simulink model "day03"  (R2026a)
settings: Solver=VariableStepAuto  StopTime=inf
libraries: simulink x1
settings Model: Creator=pete  LastModifiedBy=pete

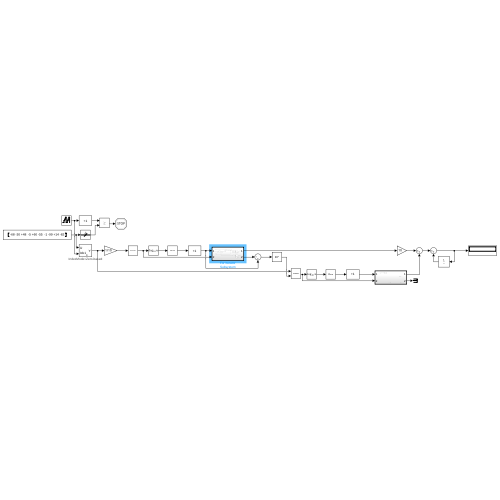
[thumbnail: Simulink's stored preview of the top-level diagram]
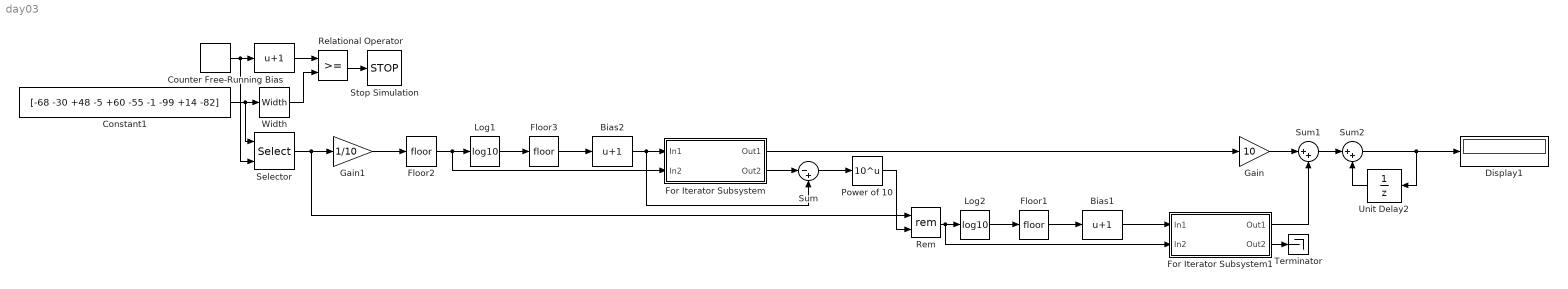
== system day03 ==
  Bias : Bias  Bias=1  SaturateOnIntegerOverflow=off
  Bias1 : Bias  Bias=1  SaturateOnIntegerOverflow=off
  Bias2 : Bias  Bias=1  SaturateOnIntegerOverflow=off
  Constant1 : Constant  Value=[-68 -30 +48 -5 +60 -55 -1 -99 +14 -82]
  Counter Free-Running : simulink/Sources/Counter Free-Running  NumBits=16  tsamp=-1
  Display1 : Display
  Floor1 : Rounding
  Floor2 : Rounding
  Floor3 : Rounding
  For Iterator Subsystem : Subsystem  TreatAsAtomicUnit=on
  For Iterator Subsystem1 : Subsystem  TreatAsAtomicUnit=on
  Gain : Gain  Gain=10
  Gain1 : Gain  Gain=1/10
  Log1 : Math  Operator=log10
  Log2 : Math  Operator=log10
  Power of 10 : Math  Operator=10^u
  Relational Operator : RelationalOperator  OutDataTypeStr=boolean  RndMeth=Simplest  InputSameDT=off
  Rem : Math  Operator=rem
  Selector : Selector  IndexMode=Zero-based  InputPortWidth=10  IndexOptions=Index vector (port)  Indices=[1 3]  OutputSizes=1
      settings: AttributesFormatString=IndexMode=%<IndexMode>
  Stop Simulation : Stop
  Sum : Sum  Inputs=|-+
  Sum1 : Sum  Inputs=|++
  Sum2 : Sum  Inputs=|++
  Terminator : Terminator
  Unit Delay2 : UnitDelay  SampleTime=-1
  Width : Width
  wires:
  Counter Free-Running/1 -> Selector/2, Bias/1
  Bias/1 -> Relational Operator/1
  Relational Operator/1 -> Stop Simulation/1
  Width/1 -> Relational Operator/2
  Constant1/1 -> Selector/1, Width/1
  Unit Delay2/1 -> Sum2/2
  Sum2/1 -> Display1/1, Unit Delay2/1
  Gain1/1 -> Floor2/1
  Log1/1 -> Floor3/1
  Floor3/1 -> Bias2/1
  Floor2/1 -> For Iterator Subsystem/2(In2), Log1/1
  Selector/1 -> Rem/1, Gain1/1
  Bias2/1 -> Sum/2, For Iterator Subsystem/1(In1)
  For Iterator Subsystem/2(Out2) -> Sum/1
  Sum/1 -> Power of 10/1
  Power of 10/1 -> Rem/2
  Log2/1 -> Floor1/1
  Floor1/1 -> Bias1/1
  Rem/1 -> For Iterator Subsystem1/2(In2), Log2/1
  Bias1/1 -> For Iterator Subsystem1/1(In1)
  For Iterator Subsystem1/2(Out2) -> Terminator/1
  Gain/1 -> Sum1/1
  For Iterator Subsystem1/1(Out1) -> Sum1/2
  Sum1/1 -> Sum2/1
  For Iterator Subsystem/1(Out1) -> Gain/1

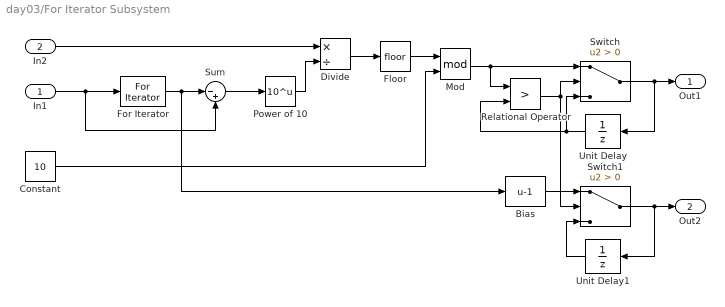
== system day03/For Iterator Subsystem ==
  In1 : Inport
  In2 : Inport  Port=2
  Bias : Bias  Bias=-1  SaturateOnIntegerOverflow=off
  Constant : Constant  Value=10
  Divide : Product  Inputs=*/
  Floor : Rounding
  For Iterator : ForIterator  ResetStates=reset  IterationSource=external
      settings: AttributesFormatString=ResetStates=%<ResetStates>
  Mod : Math  Operator=mod
  Power of 10 : Math  Operator=10^u
  Relational Operator : RelationalOperator  Operator=>  OutDataTypeStr=boolean  RndMeth=Simplest  InputSameDT=off
  Sum : Sum  Inputs=|-+
  Switch : Switch  Criteria=u2 > Threshold  SaturateOnIntegerOverflow=off  InputSameDT=off
  Switch1 : Switch  Criteria=u2 > Threshold  SaturateOnIntegerOverflow=off  InputSameDT=off
  Unit Delay : UnitDelay  SampleTime=-1
  Unit Delay1 : UnitDelay  SampleTime=-1
  Out1 : Outport
  Out2 : Outport  Port=2
  wires:
  In1/1 -> Sum/2, For Iterator/1
  For Iterator/1 -> Bias/1, Sum/1
  Sum/1 -> Power of 10/1
  In2/1 -> Divide/1
  Power of 10/1 -> Divide/2
  Divide/1 -> Floor/1
  Floor/1 -> Mod/1
  Constant/1 -> Mod/2
  Mod/1 -> Switch/1, Relational Operator/1
  Switch/1 -> Out1/1, Unit Delay/1
  Unit Delay/1 -> Switch/3, Relational Operator/2
  Switch1/1 -> Out2/1, Unit Delay1/1
  Bias/1 -> Switch1/1
  Unit Delay1/1 -> Switch1/3
  Relational Operator/1 -> Switch/2, Switch1/2

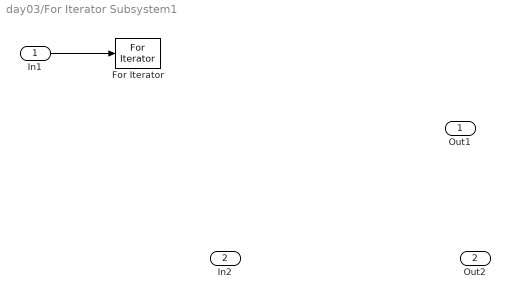
== system day03/For Iterator Subsystem1 ==
  In1 : Inport
  In2 : Inport  Port=2
  For Iterator : ForIterator  IterationSource=external
  Out1 : Outport
  Out2 : Outport  Port=2
  wires:
  In1/1 -> For Iterator/1
